simulink model "Wheel_SWC"  (R2023b)
settings: Solver=VariableStepAuto  StartTime=0.0  StopTime=10.0  RelTol=1e-3
settings Model: Creator=E8KUAVE  LastModifiedBy=E8KUAVE

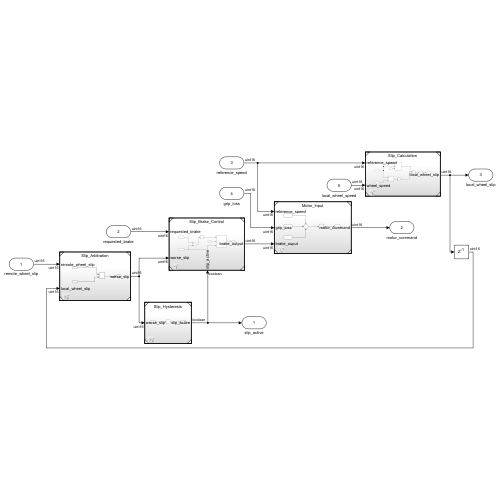
[thumbnail: Simulink's stored preview of the top-level diagram]
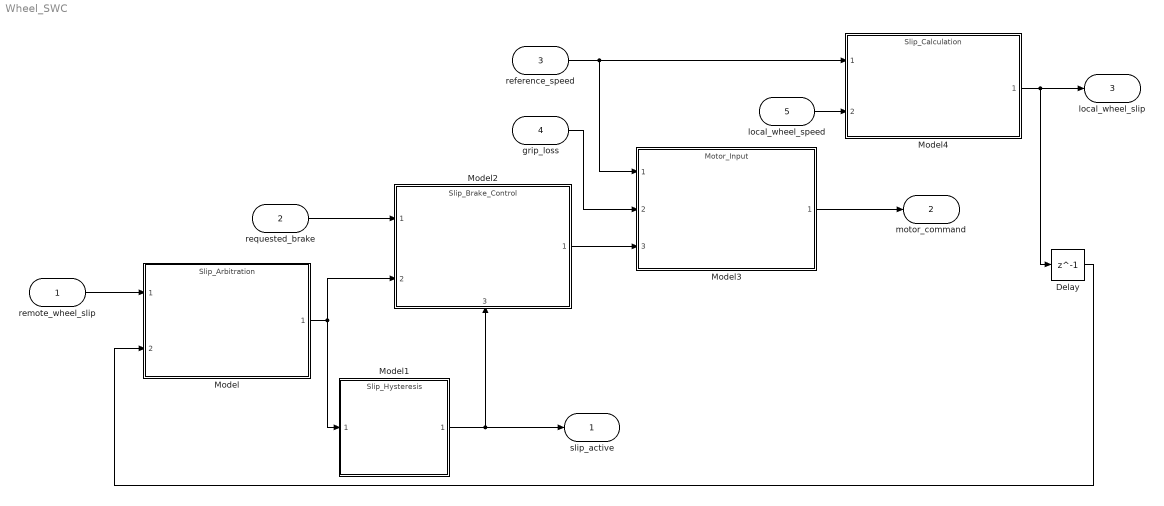
== system Wheel_SWC ==
  remote_wheel_slip : Inport  OutDataTypeStr=uint16
  requested_brake : Inport  Port=2  OutDataTypeStr=uint16
  reference_speed : Inport  Port=3  OutDataTypeStr=uint16
  grip_loss : Inport  Port=4  OutDataTypeStr=uint16
  local_wheel_speed : Inport  Port=5  OutDataTypeStr=uint16
  Delay : Delay  DelayLength=1  InitialCondition=0
  Model : ModelReference  ModelNameDialog=Slip_Arbitration.slx  SimulationMode=Normal  ModelReferenceVersion=1.1
  Model1 : ModelReference  ModelNameDialog=Slip_Hysteresis.slx  UsingDefaultArgumentValue=0,0  SimulationMode=Normal  ModelReferenceVersion=1.3
  Model2 : ModelReference  ModelNameDialog=Slip_Brake_Control.slx  SimulationMode=Normal  ModelReferenceVersion=1.2
      settings: PortSchema="{\"entries\":[{\"content\":{\"sides\":[{\"content\":{\"connectorIds\":[\"In1\",\"In2\"]},\"type\":\"ConnectorPlacement.EquallySpacedRectSide\",\"uuid\":\"43833c58-9754-4867-b06c-bf471013f472\"},{\"content\":{\"connectorIds\":[\"Out1\"],\"side\":\"RIGHT\"},\"type\":\"ConnectorPlacement.EquallySpacedRectSide\",\"uuid\":\"09d73fa1-7b80-425e-b4a4-d0713d946826\"},{\"content\":{\"side\":\"TOP\"},\"type\":\"ConnectorPlacement.EquallySpacedRectSide\",\"uuid\":\"dd602e94-9970-4c5d-a7ac-8f2a17641b15\"},{\"content\":{\"connectorIds\":[\"In3\"],\"side\":\"BOTTOM\"},\"type\":\"ConnectorPlacement.EquallySpacedRectSide\",\"uuid\":\"abe2557a-a297-41bc-8c71-4db5607c642f\"}]},\"type\":\"ConnectorPlacement.EquallySpacedConnector\",\"uuid\":\"64c77df4-7378-4fca-a84a-f77d2b83233f\"}],\"packageUris\":[\"http://schema.mathworks.com/mf0/Connector/R2020b\"],\"version\":\"1.0\"}"
  Model3 : ModelReference  ModelNameDialog=Motor_Input.slx  SimulationMode=Normal  ModelReferenceVersion=1.3
  Model4 : ModelReference  ModelNameDialog=Slip_Calculation.slx  SimulationMode=Normal  ModelReferenceVersion=1.4
  slip_active : Outport
  motor_command : Outport  Port=2
  local_wheel_slip : Outport  Port=3
  wires:
  remote_wheel_slip/1 -> Model/1
  Model/1 -> Model2/2, Model1/1
  Model1/1 -> slip_active/1, Model2/3
  requested_brake/1 -> Model2/1
  Model2/1 -> Model3/3
  reference_speed/1 -> Model4/1, Model3/1
  Model3/1 -> motor_command/1
  local_wheel_speed/1 -> Model4/2
  grip_loss/1 -> Model3/2
  Model4/1 -> Delay/1, local_wheel_slip/1
  Delay/1 -> Model/2
